simulink model "metronomo10"  (Simulink 8.1)
settings: Solver=ode45  StartTime=0.0  StopTime=10.0  RelTol=1e-6
values from neighbouring files (symbols this model uses):
  beta = .001    (= 0.001)    [Ex10.m]    (also in Ex4.m = 0.1; Ex5.m = 0.1; Ex6.m = b(i); Ex6_2.m = b(i))
  g = 10    [Ex10.m]    (also in Ex4.m; Ex5.m; Ex6.m; Ex6_2.m)
  J = 1/3*M*L^2 + m*l^2    (= 0.0168738257353)    [Ex10.m]    (also in Ex4.m = 0.0413333333333; Ex5.m = 0.0413333333333; Ex6.m = 0.0413333333333; Ex6_2.m = 0.0413333333333)
  k = 1    [Ex10.m]    (also in Ex4.m = 5; Ex5.m = 5; Ex6.m = 5; Ex6_2.m = 5)
  L = .2    (= 0.2)    [Ex10.m]    (also in Ex4.m = 0.4; Ex5.m = 0.4; Ex6.m = 0.4; Ex6_2.m = 0.4)
  l = l2    (= 0.176298)    [Ex10.m]    (also in Ex4.m = 0.3; Ex5.m = 0.3; Ex6.m = 0.3; Ex6_2.m = 0.3)
  M = .1    (= 0.1)    [Ex10.m]    (also in Ex4.m; Ex5.m; Ex6.m; Ex6_2.m)
  m = 0.5    [Ex10.m]    (also in Ex4.m = 0.4; Ex5.m = 0.4; Ex6.m = 0.4; Ex6_2.m = 0.4)
  w = 1.047    [Ex10.m]    (also in Ex9.m = 0.524)
  x0 = [x01 0]    [Ex10.m]    (also in Ex4.m = [pi/16 0]; Ex5.m = [pi/16 0]; Ex6.m = [pi/16 0]; Ex6_2.m = [x01i(c1) x02i(c2)])
  x01 = pi/16    (= 0.196349540849)    [Ex10.m]
settings Model: Creator=g  LastModifiedBy=Diogo Bras

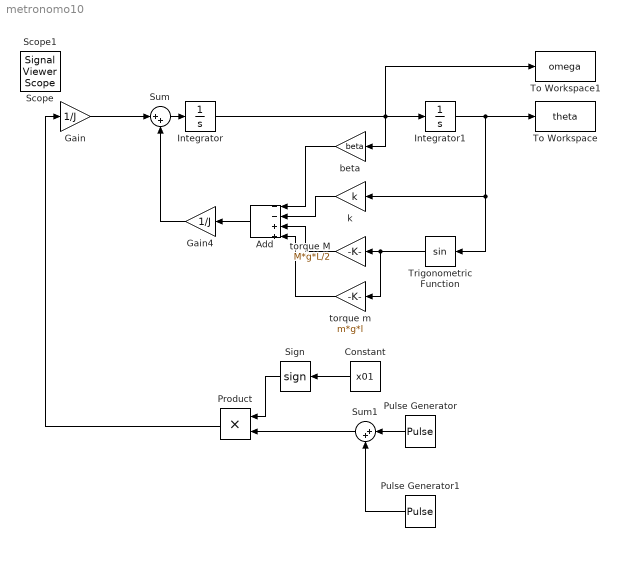
== system metronomo10 ==
  Add : Sum  Inputs=--++
  Constant : Constant  Value=x01
  Gain : Gain  Gain=1/J
  Gain4 : Gain  Gain=1/J
  Integrator : Integrator  InitialCondition=x0(2)
  Integrator1 : Integrator  InitialCondition=x0(1)
  Product : Product
  Pulse Generator : DiscretePulseGenerator  PulseType=Time based  Amplitude=J/2  Period=(2*pi/w)  PulseWidth=5  PhaseDelay=(1/4)*(2*pi/w)
  Pulse Generator1 : DiscretePulseGenerator  PulseType=Time based  Amplitude=-J/2  Period=(2*pi/w)  PulseWidth=5  PhaseDelay=(3/4)*(2*pi/w)
  Sign : Signum
  Sum : Sum  Inputs=|++
  Sum1 : Sum  Inputs=|++
  To Workspace : ToWorkspace  VariableName=theta  SampleTime=-1
  To Workspace1 : ToWorkspace  VariableName=omega  SampleTime=-1
  Trigonometric Function : Trigonometry
  beta : Gain  Gain=beta
  k : Gain  Gain=k
  torque M : Gain  Gain=M*g*L/2
  torque m : Gain  Gain=m*g*l
  Scope : SignalViewerScope  IOType=viewer  RefreshTime=0.035000
  Scope1 : SignalViewerScope  IOType=viewer  RefreshTime=0.035000
  wires:
  Integrator/1 -> Integrator1/1, beta/1, To Workspace1/1
  Trigonometric Function/1 -> torque M/1, torque m/1
  Integrator1/1 -> Trigonometric Function/1, k/1, To Workspace/1
  beta/1 -> Add/1
  k/1 -> Add/2
  torque M/1 -> Add/3
  torque m/1 -> Add/4
  Add/1 -> Gain4/1
  Gain4/1 -> Sum/2
  Sum/1 -> Integrator/1
  Gain/1 -> Sum/1
  Pulse Generator/1 -> Sum1/1
  Pulse Generator1/1 -> Sum1/2
  Sign/1 -> Product/1
  Sum1/1 -> Product/2
  Constant/1 -> Sign/1
  Product/1 -> Gain/1
